simulink model "Horizontal_Turn_Symmetric"  (R2021b)
settings: Solver=ode4  StartTime=0.0  StopTime=50  FixedStep=0.01  RelTol=1e-1
values from neighbouring files (symbols this model uses):
  alpha_ = atan(y(3)/y(1))    [Trim_sym.m]    (also in Trim_sym.mat = 0.357010867724)
  b = 2.8956    [Constants_sym.m]    (also in Trim_sym_main.m)
  cbar = 0.18994    [Constants_sym.m]    (also in Trim_sym_main.m)
  Cprop = 1    [Constants_sym.m]    (also in Trim_sym_main.m)
  d2r = pi/180    (= 0.0174532925199)    [Constants_sym.m]    (also in Trim_sym.m; Trim_sym_main.m)
  g = 9.81    [Constants_sym.m]    (also in Trim_sym_main.m)
  Ixx = 0.8244    [Constants_sym.m]    (also in Trim_sym_main.m)
  Ixz = 0.1204    [Constants_sym.m]    (also in Trim_sym_main.m)
  Iyy = 1.135    [Constants_sym.m]    (also in Trim_sym_main.m)
  Izz = 1.759    [Constants_sym.m]    (also in Trim_sym_main.m)
  Kmotor = 80    [Constants_sym.m]    (also in Trim_sym_main.m)
  m = 13.5    [Constants_sym.m]    (also in Trim_sym_main.m)
  q = 0    [Trim_sym.m]
  qbar = 0.5*rho*V^2    [Constants_sym.m]    (also in Trim_sym_main.m = 186.625322459)
  r = 0    [Trim_sym.m]
  r2d = 180/pi    (= 57.2957795131)    [Constants_sym.m]    (also in Trim_sym.m; Trim_sym_main.m)
  rho = p_atm/(287*T_atm)    [Constants_sym.m]    (also in Trim_sym_main.m = 1.44533597728)
  S = 0.55    [Constants_sym.m]    (also in Trim_sym_main.m)
  Sprop = 0.2027    [Constants_sym.m]    (also in Trim_sym_main.m)
  V = 16.07    [Trim_sym.mat]    (also in Trim_sym_main.m)
undefined symbols (not defined in the file or in its folder): F, Light, MIL, sigbuilder_block
libraries: aerolibwind2 x3, simulink x1, slpidlib x1, sharedtransform x1
(part 1 of 2)
settings Model: Creator=Prateek  LastModifiedBy=piyus
settings SolverCC: MaxConsecutiveMinStep=100  AlgebraicLoopSolver=LineSearch
settings DataIOCC: ReturnWorkspaceOutputs=off
settings DebuggingCC: SFMachineParentedDataDiag=warning  ArithmeticOperatorsInVariantConditions=warning
settings SFSimCC: CustomCodeUndefinedFunction=UseInterfaceOnly

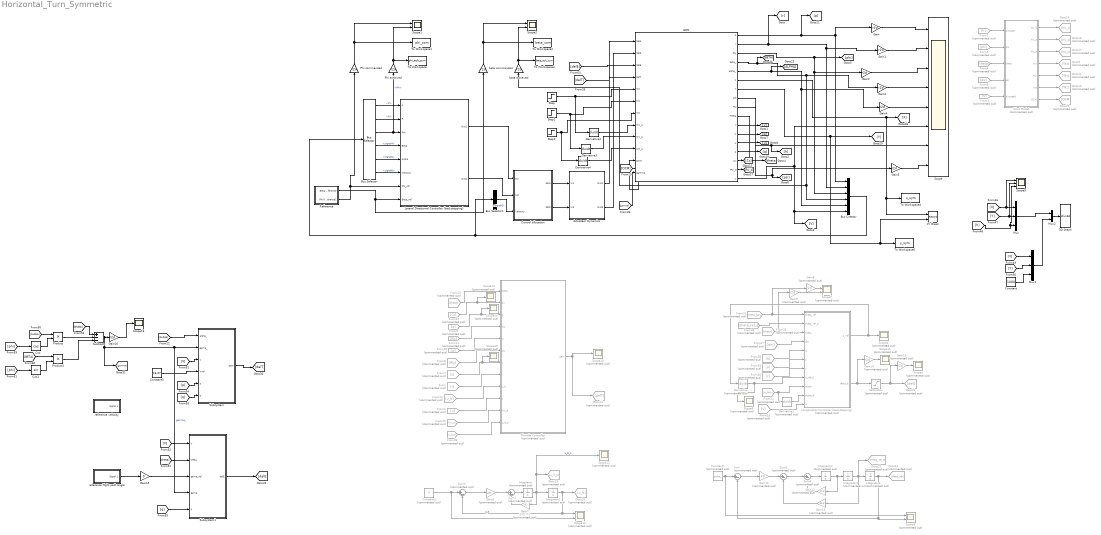
== system Horizontal_Turn_Symmetric ==
  3D Graph : S-Function  LoadFcn=if exist('sfun3d','file'), sfun3d([],[],[],'LoadBlock'); end  FunctionName=sfun3d  Parameters=ax,T,np,cp,gd,ls,mk,mx,hd,tb  SFunctionDeploymentMode=off  EnableBusSupport=off  mask(3D Graph){np=2, ax=[0 500 -20 300 500 3000], mx=1e4, T=0.01, cp=[500 -300 700], gd=on, hd=on, tb=off, ls=-, mk=.}
      mask prompts: np "Number of moving points (lines)"; ax "Range: [xmin xmax  ymin ymax zmin zmax]"; mx "Max number of points in each line"; T "Sampling Time"; cp "Camera position (use [0 0 1] for 2D XY view)"; gd "Grid (on|off)"; hd "HeadMarkers (on|off)"; tb "Toolbar (on|off)"; ls "LineStyle"; mk "LineMarker"
      mask help:
      | This block plots the position of several points in the XYZ space. The input contains the coordinates of all the points (x1,y1,z1,x2,y2,z2,...).
      | The number of moving points (lines), the XYZ ranges, sampling time, camera position, and grid (among other things) can be set as mask parameters.
      settings: CopyFcn=if exist('sfun3d','file'), sfun3d([],[],[],'CopyBlock'); end  DeleteFcn=if exist('sfun3d','file'), sfun3d([],[],[],'DeleteBlock'); end  NameChangeFcn=if exist('sfun3d','file'), sfun3d([],[],[],'NameChange'); end
      mask Help:
      | This block plots the position of several points in the XYZ space. The input contains the coordinates of all the points (x1,y1,z1,x2,y2,z2,...).
      | The number of moving points (lines), the XYZ ranges, sampling time, camera position, and grid (among other things) can be set as mask parameters.
      mask TypeOptions ls: - | -- | : | -. | none
      mask TypeOptions mk: none | . | + | o | * | x | square | diamond | v | ^ | > | < | pentagram | hexagram
      mask Display: plot([.05 .95 .95 .05 .05],[.45 .45 .95 .95 .45], 0.5+cos(0:0.1:2*pi)*0.3,0.7+sin(0:0.1:2*pi)*0.2)
  Actuataor Dynamics : Subsystem
  Bus Creator : BusCreator  Inputs=6
  Bus Selector : BusSelector  OutputSignals=P,R,Phi,signal4,signal5,signal6
  Bus Selector1 : BusSelector  OutputSignals=signal6
  Constant : Constant  Value=1000
  Constant1 : Constant  Commented=on  Value=alpha_
  Constant2 : Constant  Commented=on  Value=V
  Constant3 : Constant  Value=16.07
  Control allocation : Subsystem
  Cos : Trigonometry  Operator=cos
  Cos1 : Trigonometry
  Derivative : Derivative  Commented=on
  Derivative1 : Derivative  Commented=on
  Derivative2 : Derivative
  Derivative3 : Derivative
  Derivative4 : Derivative
  EOM : Subsystem
  From : From  Commented=on  GotoTag=r
  From1 : From  Commented=on  GotoTag=u
  From10 : From  Commented=on  GotoTag=w
  From11 : From  Commented=on  GotoTag=Wz
  From12 : From  Commented=on  GotoTag=Cx
  From13 : From  Commented=on  GotoTag=theta
  From14 : From  Commented=on  GotoTag=u_b
  From15 : From  Commented=on  GotoTag=Wx_p
  From2 : From  Commented=on  GotoTag=h
  From23 : From  Commented=on  GotoTag=u_b_p
  From24 : From  Commented=on  GotoTag=ALPHA
  From26 : From  Commented=on  GotoTag=theta
  From27 : From  Commented=on  GotoTag=phi
  From28 : From  Commented=on  GotoTag=q
  From29 : From  Commented=on  GotoTag=p
  From3 : From  Commented=on  GotoTag=V
  From30 : From  Commented=on  GotoTag=r
  From31 : From  Commented=on  GotoTag=theta_bar
  From33 : From  Commented=on  GotoTag=V
  From34 : From  Commented=on  GotoTag=theta_ref_d
  From4 : From  Commented=on  GotoTag=theta
  From5 : From  Commented=on  GotoTag=phi
  From6 : From  Commented=on  GotoTag=psi
  From7 : From  Commented=on  GotoTag=v
  From8 : From  Commented=on  GotoTag=Wy
  From9 : From  Commented=on  GotoTag=q
  Gain{,1..5,16} (7 alike) : Gain  Gain=r2d
  Gain{8..10,14} (4 alike) : Gain  Commented=on  Gain=r2d
  Gain11 : Gain  Commented=on  Gain=49
  Gain12 : Gain  Commented=on  Gain=10.8
  Gain13 : Gain  Commented=on  Gain=58.8
  Gain15 : Gain  Gain=0
  Gain6 : Gain  Commented=on  Gain=49
  Gain7 : Gain  Commented=on  Gain=2*0.7*7
  Goto11 : Goto  Commented=on  GotoTag=Wy
  Goto13 : Goto  Commented=on  GotoTag=delT
  Goto14 : Goto  Commented=on  GotoTag=Wx_p
  Goto15 : Goto  Commented=on  GotoTag=Wz
  Goto16 : Goto  Commented=on  GotoTag=Wy_p
  Goto17 : Goto  Commented=on  GotoTag=Wz_p
  Goto18 : Goto  Commented=on  GotoTag=u_b
  Goto19 : Goto  Commented=on  GotoTag=u_b_p
  Goto20 : Goto  Commented=on  GotoTag=DCM
  Goto23 : Goto  Commented=on  GotoTag=delE
  Goto24 : Goto  Commented=on  GotoTag=theta_bar
  Goto25 : Goto  Commented=on  GotoTag=theta_ref_d
  Goto9 : Goto  Commented=on  GotoTag=Wx
  Integrator{,2..4} (4 alike) : Integrator  Commented=on
  Integrator1 : Integrator  Commented=on  InitialCondition=19.5
  Lateral Directional Controller (backstepping) : Subsystem
  Longitudinal Controller (backstepping) : MATLAB Function  Commented=on  TreatAsAtomicUnit=on
  Mux : Mux  Inputs=3
  Mux1 : Mux  Inputs=3
  Mux2 : Mux  Inputs=2
  Phi acheived : Gain  Gain=r2d
  Phi commanded : Gain  Gain=r2d
  Product : Product
  Product1 : Product
  Reference : Subsystem
  Saturation : Saturate  Commented=on  UpperLimit=30*d2r  LowerLimit=-(30*d2r)
  Scope : Scope  NumInputPorts=8
  Scope1 : Scope  NumInputPorts=2
  Scope{3..4,6,10..11,13..15,19} (9 alike) : Scope  Commented=on
  Scope12 : Scope  Commented=on  NumInputPorts=2
  Scope16 : Scope
  Scope2 : Scope  NumInputPorts=2
  Scope5 : Scope  NumInputPorts=3
  Scope7 : Scope  Commented=on  NumInputPorts=2
  Scope8 : Scope  Commented=on  NumInputPorts=2
  Step : Step  Time=0  After=0  SampleTime=0
  Step1 : Step  Time=0  After=0  SampleTime=0
  Step2 : Step  Time=0  After=3  SampleTime=0
  Subsystem : Subsystem
  Subsystem1 : Subsystem
  Subtract : Sum  Inputs=+--
  Sum{,1..4} (5 alike) : Sum  Commented=on  Inputs=|+-
  Throttle Controller : Subsystem  Commented=on
  To Workspace : ToWorkspace  VariableName=phi_ach_sym  SampleTime=-1
  To Workspace1 : ToWorkspace  VariableName=phi_com  SampleTime=-1
  To Workspace2 : ToWorkspace  VariableName=beta_com  SampleTime=-1
  To Workspace3 : ToWorkspace  VariableName=beta_ach_sym  SampleTime=-1
  To Workspace4 : ToWorkspace  VariableName=x_sym  SampleTime=-1
  To Workspace5 : ToWorkspace  VariableName=y_sym  SampleTime=-1
  "Wind Model " : Subsystem  Commented=on
  XY Graph : Record  FileSettingsInternal="{\"entries\":[{\"content\":{\"excelSettings\":{\"content\":{},\"type\":\"Streamout.ExcelSettings\"}},\"type\":\"Streamout.FileSettingStorage\",\"uuid\":\"f48354ea-9da4-4102-8cec-34de0f807aaf\"}],\"packageUris\":[\"http://schema.mathworks.com/mf0/streamout_blocks/R2020a\"],\"version\":\"1.0\"}"  Layout=[1 1]  SignalsInternal="{\"entries\":[{\"content\":{\"signals\":[{\"content\":{\"blockPath\":[\"Horizontal_Turn_Symmetric/XY Graph\"],\"channel\":[],\"dimensions\":[1],\"domain\":\"Horizontal_Turn_Symmetric/XY Graph\",\"lineColor\":\"#a2142f\",\"plots\":[1],\"port\":1,\"sid\":[],\"signalID\":54,\"signalName\":\"EOM:6\"},\"type\":\"RecordBlkView.Signal\",\"uuid\":\"b83f61b6-62b6-4807-96de-0ee58c6a34da\"},{\"content\":{\"blockPath\":[\"Horizontal_Turn_Symmetric/XY Graph\"],\"channel\":[],\"dimensions\":[1],\"domain\":\"Horizontal_Turn_Symmetric/XY Graph\",\"lineColor\":\"#139fff\",\"plots\":[1],\"port\":2,\"sid\":[],\"signalID\":57,\"signalName\":\"EOM:7\"},\"type\":\"RecordBlkView.Signal\",\"uuid\":\"4337f21f-c38c-4e87-a719-4f27d7101128\"}]},\"type\":\"RecordBlkView.InputSignals\",\"uuid\":\"b9ba9dc8-fadb-49a6-9e4e-9d1384d51f42\"}],\"packageUris\":[\"http://schema.mathworks.com/mf0/streamout_blocks/R2020a\"],\"version\":\"1.0\"}"  VisualizationBindings="{\"xyplotplugin\":{\"info\":[{\"series\":[{\"bindingParametersList\":[{\"parameter\":\"X-Axis\",\"signalID\":54,\"signalName\":\"EOM:6\"},{\"parameter\":\"Y-Axis\",\"signalID\":57,\"signalName\":\"EOM:7\"}],\"seriesID\":61385}],\"subplotID\":1}]}}"  CompatibilityTag=XY  st=-1
  beta achieved : Gain  Gain=r2d
  beta commanded : Gain  Gain=r2d
  reference flight path angle : Subsystem  Tag=STV Subsys  LoadFcn=sigbuilder_block('load');  StartFcn=sigbuilder_block('start');  StopFcn=sigbuilder_block('stop');  ClipboardFcn=sigbuilder_block('clipboard');  mask(Sigbuilder block){tuvar=[0:10]}
      mask help: Simulink:masks:SigbuilderBlock_MD
      mask init:
      | if ~strcmp(get_param(bdroot(gcbh),'SimulationStatus'),'stopped') tuvar = sigbuilder_block('maskInit'); end
      settings: CopyFcn=sigbuilder_block('copy');  DeleteFcn=sigbuilder_block('delete');  ModelCloseFcn=sigbuilder_block('modelClose');  PreSaveFcn=sigbuilder_block('preSave');  PauseFcn=sigbuilder_block('pause');  ContinueFcn=sigbuilder_block('continue');  NameChangeFcn=sigbuilder_block('namechange');  OpenFcn=sigbuilder_block('open',[5.4 0 1141.2 552.6 ]);  CloseFcn=sigbuilder_block('close');
      mask Display: plot(0, 0, 100, 100,[2, 2, 32, 32, 2], [68, 8, 8, 68, 68],[32, 2], [38, 38], [32, 19, 2],[53, 60, 44], [32, 17, 17, 2],[16, 16, 31, 31]);txt = getActiveGroup(gcbh);text(2, 100, txt,'verticalAlignment', 'top');
  reference velocity : Subsystem  Tag=STV Subsys  LoadFcn=sigbuilder_block('load');  StartFcn=sigbuilder_block('start');  StopFcn=sigbuilder_block('stop');  ClipboardFcn=sigbuilder_block('clipboard');  mask(Sigbuilder block){tuvar=[0:10]}
      mask help: Simulink:masks:SigbuilderBlock_MD
      mask init:
      | if ~strcmp(get_param(bdroot(gcbh),'SimulationStatus'),'stopped') tuvar = sigbuilder_block('maskInit'); end
      settings: CopyFcn=sigbuilder_block('copy');  DeleteFcn=sigbuilder_block('delete');  ModelCloseFcn=sigbuilder_block('modelClose');  PreSaveFcn=sigbuilder_block('preSave');  PauseFcn=sigbuilder_block('pause');  ContinueFcn=sigbuilder_block('continue');  NameChangeFcn=sigbuilder_block('namechange');  OpenFcn=sigbuilder_block('open',[5.4 0 1141.2 552.6 ]);  CloseFcn=sigbuilder_block('close');
      mask Display: plot(0, 0, 100, 100,[2, 2, 32, 32, 2], [68, 8, 8, 68, 68],[32, 2], [38, 38], [32, 19, 2],[53, 60, 44], [32, 17, 17, 2],[16, 16, 31, 31]);txt = getActiveGroup(gcbh);text(2, 100, txt,'verticalAlignment', 'top');
  wires:
  Bus Creator/1 -> Bus Selector/1, Bus Selector1/1
  Control allocation/1(delA) -> Actuataor Dynamics/1(In1)
  Control allocation/2(delR) -> Actuataor Dynamics/2(In3)
  Lateral Directional Controller (backstepping)/1(Out1) -> Control allocation/1(MX)
  Phi commanded/1 -> To Workspace1/1, Scope1/1
  Lateral Directional Controller (backstepping)/2(Out2) -> Control allocation/2(MZ)
  Reference/1(Beta Reference) -> beta commanded/1, Lateral Directional Controller (backstepping)/8(Beta_ref)
  Phi acheived/1 -> Scope1/2, To Workspace/1
  beta commanded/1 -> To Workspace2/1, Scope2/1
  Gain3/1 -> Scope/4
  Gain4/1 -> Scope/5
  Gain/1 -> Scope/1
  Gain1/1 -> Scope/2
  Gain2/1 -> Scope/3
  Bus Selector1/1 -> Control allocation/3(Velocity)  "<signal6>"
  Bus Selector/1 -> Lateral Directional Controller (backstepping)/1(P)  "<P>"
  Bus Selector/2 -> Lateral Directional Controller (backstepping)/2(R)  "<R>"
  Bus Selector/3 -> Phi acheived/1, Lateral Directional Controller (backstepping)/3(PHI)  "<Phi>"
  Bus Selector/4 -> Lateral Directional Controller (backstepping)/4(Beta)  "<signal4>"
  Bus Selector/5 -> Lateral Directional Controller (backstepping)/5(Alpha)  "<signal5>"
  Bus Selector/6 -> Lateral Directional Controller (backstepping)/6(Velocity)  "<signal6>"
  Gain5/1 -> Scope/8
  Actuataor Dynamics/1(Out1) -> EOM/1(delA)
  Actuataor Dynamics/2(Out6) -> EOM/2(delR)
  [delT] -> EOM/4(delT)
  EOM/1(p) -> [p], Gain/1, Bus Creator/1
  EOM/2(r) -> Bus Creator/2, Gain1/1, [r]
  EOM/3(Phi) -> [phi], Bus Creator/3, Gain2/1
  EOM/4(beta_) -> [BETA], Bus Creator/4, beta achieved/1, Gain3/1
  EOM/5(alpha_) -> [ALPHA], Bus Creator/5, Gain4/1
  EOM/17(V) -> Scope/6, [V], Bus Creator/6
  EOM/6(X) -> [X], To Workspace4/1, XY Graph/1
  EOM/8(Alt) -> [h], Scope/7
  EOM/9(Psi) -> Gain5/1, [psi]
  beta achieved/1 -> Scope2/2, To Workspace3/1
  EOM/11(v) -> [v]
  EOM/10(Theta) -> [theta]
  EOM/12(w) -> [w]
  EOM/13(u) -> [u]
  EOM/14(q) -> [q]
  EOM/15(Cx) -> [Cx]
  From13/1 -> Throttle Controller/1(theta)
  From12/1 -> Scope14/1, Throttle Controller/2(Cx)
  From9/1 -> Scope15/1, Throttle Controller/3(q)
  From11/1 -> Throttle Controller/4(Wz)
  From10/1 -> Throttle Controller/5(w)
  From8/1 -> Throttle Controller/6(Wy)
  From7/1 -> Throttle Controller/7(v), Scope19/1
  From/1 -> Throttle Controller/8(r)
  From14/1 -> Throttle Controller/9(u_b)
  From1/1 -> Throttle Controller/10(u)
  From15/1 -> Throttle Controller/11(Wx_p)
  Throttle Controller/1(delT) -> Goto13/1, Scope10/1
  Step/1 -> Derivative2/1, EOM/5(Wx)
  Step1/1 -> Derivative3/1, EOM/6(Wy)
  Derivative2/1 -> EOM/8(Wx_p)
  Derivative3/1 -> EOM/9(Wy_p)
  Derivative4/1 -> EOM/10(Wz_p)
  Constant2/1 -> Scope12/2, Sum1/1
  Integrator1/1 -> Goto18/1, Sum1/2, Scope12/1  "u_b"
  Sum1/1 -> Gain6/1
  Gain6/1 -> Sum2/1
  Sum2/1 -> Integrator/1
  Integrator/1 -> Scope13/1, Goto19/1, Integrator1/1, Gain7/1  "u_b_p"
  Gain7/1 -> Sum2/2
  From23/1 -> Throttle Controller/12(u_b_p)
  [DCM] -> EOM/11(DCM)
  From2/1 -> "Wind Model "/1(Altitude)
  From5/1 -> "Wind Model "/2(phi)
  From4/1 -> "Wind Model "/3(theta)
  From6/1 -> "Wind Model "/4(psi)
  From3/1 -> "Wind Model "/5(Airspeed)
  "Wind Model "/1(Wx_p) -> Goto14/1
  "Wind Model "/2(Wy_p) -> Goto16/1
  "Wind Model "/3(Wz_p) -> Goto17/1
  EOM/7(Y) -> XY Graph/2, To Workspace5/1, [Y]
  "Wind Model "/4(Wx) -> Goto9/1
  "Wind Model "/5(Wy) -> Goto11/1
  "Wind Model "/6(Wz) -> Goto15/1
  "Wind Model "/7(DCM) -> Goto20/1
  From26/1 -> Longitudinal Controller (backstepping)/3(theta), Gain9/1
  From27/1 -> Longitudinal Controller (backstepping)/4(phi)
  From28/1 -> Longitudinal Controller (backstepping)/5(q)
  From29/1 -> Longitudinal Controller (backstepping)/6(p)
  From30/1 -> Longitudinal Controller (backstepping)/7(r)
  Longitudinal Controller (backstepping)/1(q_ref) -> Scope4/1, Derivative/1
  From31/1 -> Longitudinal Controller (backstepping)/1(theta_ref), Gain8/1
  From33/1 -> Longitudinal Controller (backstepping)/11(V)
  [delE] -> EOM/3(delE)
  Derivative/1 -> Scope6/1, Longitudinal Controller (backstepping)/8(q_ref_d)
  Saturation/1 -> Goto23/1, Gain10/1
  Gain9/1 -> Scope7/2
  Gain8/1 -> Scope7/1
  Gain10/1 -> Scope3/1
  Constant1/1 -> Sum/1, Scope8/1
  Integrator4/1 -> Goto24/1, Sum/2, Scope8/2
  Sum/1 -> Gain11/1
  Gain11/1 -> Sum3/1
  Sum3/1 -> Sum4/1
  Sum4/1 -> Integrator2/1
  Integrator2/1 -> Gain12/1, Integrator3/1
  Integrator3/1 -> Goto25/1, Gain13/1, Integrator4/1
  Gain12/1 -> Sum4/2
  Gain13/1 -> Sum3/2
  From34/1 -> Longitudinal Controller (backstepping)/2(theta_ref_d)
  EOM/16(Psi_d) -> [Psi_d]
  From24/1 -> Derivative1/1, Longitudinal Controller (backstepping)/9(alpha)
  Derivative1/1 -> Longitudinal Controller (backstepping)/10(alpha_d)
  Mux/1 -> Mux2/1
  [Y] -> Scope5/2, Mux/2
  [X] -> Scope5/1, Mux/1
  [h] -> Scope5/3, Mux/3
  [X] -> Mux1/1
  [Y] -> Mux1/2
  Constant/1 -> Mux1/3
  Mux1/1 -> Mux2/2
  Mux2/1 -> 3D Graph/1
  Longitudinal Controller (backstepping)/2(delta_e) -> Gain14/1, Saturation/1
  Gain14/1 -> Scope11/1
  [ALPHA] -> Subsystem/1(alpha_)
  [V] -> Subsystem/3(V)
  Subsystem/1(delT) -> [delT]
  [V] -> Subsystem1/1(V)
  [theta] -> Subsystem1/2(theta)
  [q] -> Subsystem1/5(q)
  Subsystem1/1(delE) -> [delE]
  [theta] -> Subtract/1
  [ALPHA] -> Product/1
  [p] -> Subsystem/5(p)
  [q] -> Subsystem/6(q)
  reference flight path angle/1(Signal 1) -> Gain15/1
  Cos/1 -> Product/2
  Product/1 -> Subtract/2
  [phi] -> Cos/1
  [BETA] -> Product1/1
  Cos1/1 -> Product1/2
  [phi] -> Cos1/1
  Product1/1 -> Subtract/3
  Gain16/1 -> Scope16/1
  Subtract/1 -> [gamma], Subsystem1/4(gama), Subsystem/2(gama_), Gain16/1  "gamma_"
  Gain15/1 -> Subsystem1/3(gama_ref)
  Constant3/1 -> Subsystem/4(Vref)
  [gamma] -> EOM/12(gamma)
  Reference/2(Phi Reference1) -> Phi commanded/1, Lateral Directional Controller (backstepping)/7(Phi_ref)
  Step2/1 -> Derivative4/1, EOM/7(Wz)

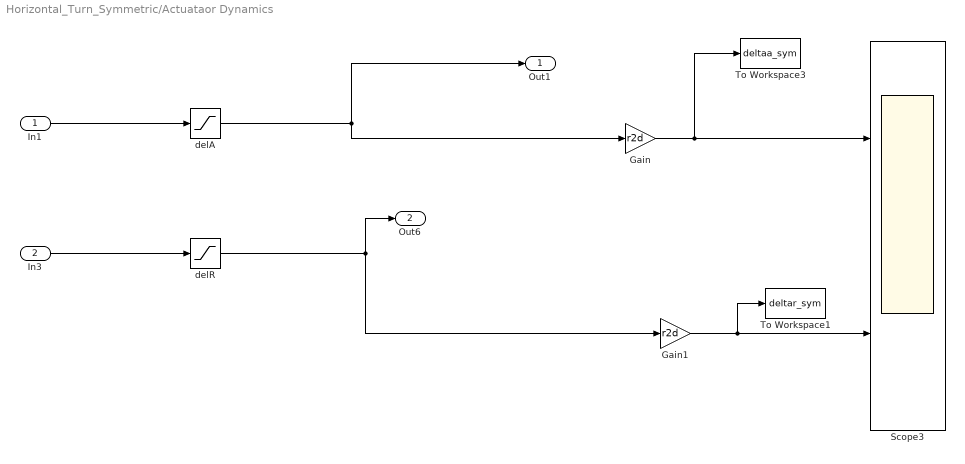
== system Horizontal_Turn_Symmetric/Actuataor Dynamics ==
  In1 : Inport
  In3 : Inport  Port=2
  Gain : Gain  Gain=r2d
  Gain1 : Gain  Gain=r2d
  Scope3 : Scope  NumInputPorts=2
  To Workspace1 : ToWorkspace  VariableName=deltar_sym  SampleTime=-1
  To Workspace3 : ToWorkspace  VariableName=deltaa_sym  SampleTime=-1
  delA : Saturate  UpperLimit=20*d2r  LowerLimit=-20*d2r
  delR : Saturate  UpperLimit=30*d2r  LowerLimit=-30*d2r
  Out1 : Outport  VectorParamsAs1DForOutWhenUnconnected=off
  Out6 : Outport  Port=2  VectorParamsAs1DForOutWhenUnconnected=off
  wires:
  delR/1 -> Gain1/1, Out6/1
  In1/1 -> delA/1
  In3/1 -> delR/1
  Gain/1 -> To Workspace3/1, Scope3/1
  Gain1/1 -> To Workspace1/1, Scope3/2
  delA/1 -> Gain/1, Out1/1

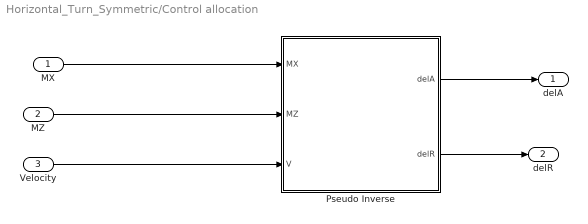
== system Horizontal_Turn_Symmetric/Control allocation ==
  MX : Inport
  MZ : Inport  Port=2
  Velocity : Inport  Port=3
  Pseudo Inverse : MATLAB Function  TreatAsAtomicUnit=on
  delA : Outport  VectorParamsAs1DForOutWhenUnconnected=off
  delR : Outport  Port=2  VectorParamsAs1DForOutWhenUnconnected=off
  wires:
  Velocity/1 -> Pseudo Inverse/3(V)
  MX/1 -> Pseudo Inverse/1(MX)
  MZ/1 -> Pseudo Inverse/2(MZ)
  Pseudo Inverse/1(delA) -> delA/1
  Pseudo Inverse/2(delR) -> delR/1

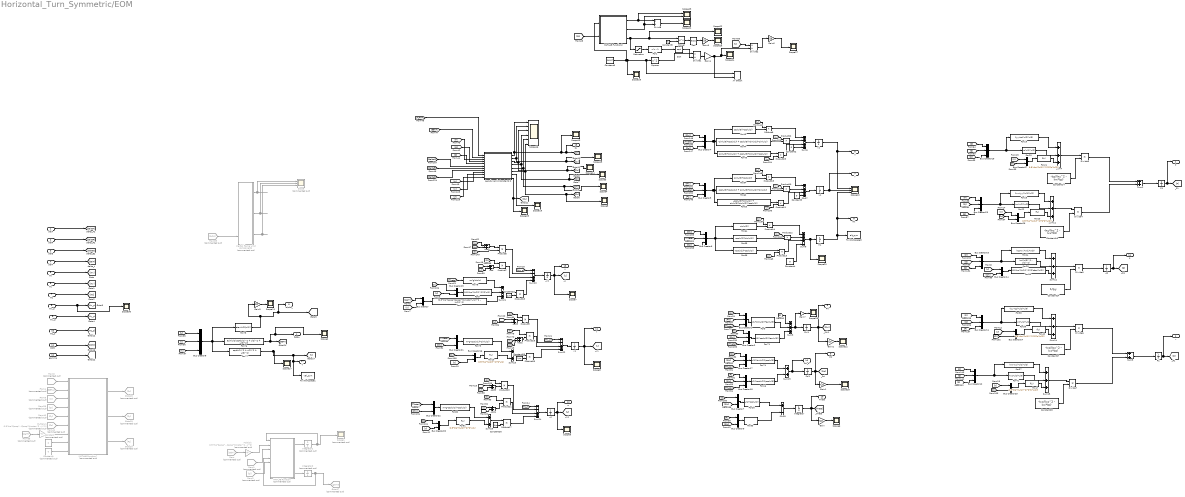
== system Horizontal_Turn_Symmetric/EOM ==
  delA : Inport
  delR : Inport  Port=2
  delE : Inport  Port=3
  delT : Inport  Port=4
  Wx : Inport  Port=5
  Wy : Inport  Port=6
  Wz : Inport  Port=7
  Wx_p : Inport  Port=8
  Wy_p : Inport  Port=9
  Wz_p : Inport  Port=10
  DCM : Inport  Port=11
  gamma : Inport  Port=12
  Add{,1..5} (6 alike) : Sum
  Aerodynamic Constants 2 : MATLAB Function  TreatAsAtomicUnit=on
  Bus Creator{,7,9,14..16,20..22,24..27} (13 alike) : BusCreator  Inputs=2
  Bus Creator{1..4,6,8,10..12,17..19,23} (13 alike) : BusCreator  Inputs=3
  Constant : Constant  Commented=on  Value=0
  Constant1 : Constant  Commented=on  Value=0
  Constant14 : Constant  Value=-Izz/(Ixz^2 - Ixx*Izz)
  Constant16 : Constant  Value=-Ixz/(Ixz^2 - Ixx*Izz)
  Constant2 : Constant  Value=0
  Constant23 : Constant  Value=1/m
  Constant24 : Constant  Value=1/Iyy
  Constant25 : Constant  Value=1/m
  Constant26 : Constant  Value=1/m
  Constant27 : Constant  Value=-Ixz/(Ixz^2 - Ixx*Izz)
  Constant28 : Constant  Value=-Ixx/(Ixz^2 - Ixx*Izz)
  Constant3 : Constant  Value=0
  Constant4 : Constant  Value=0
  Constant5 : Constant  Value=-1
  Constant6 : Constant  Value=16.07
  Cos : Trigonometry  Operator=acos
  Divide : Product  Inputs=*/
  Divide1 : Product  Inputs=*/
  Divide2 : Product  Inputs=*/
  Divide{3..7} (5 alike) : Product  Inputs=**
  Fcn1 : Fcn  Expr=u*u - 1
  Fcn10 : Fcn  Expr=0.5*rho*((u(2))^2)*S*u(1)
  Fcn16 : Fcn  Expr=u(1)*cos(u(2))/cos(u(3))
  Fcn18 : Fcn  Expr=(Ixx-Iyy)*u(1)*u(2)
  Fcn19 : Fcn  Expr=(Iyy-Izz)*u(2)*u(3)
  Fcn20 : Fcn  Expr=Ixz*u(1)*u(2)
  Fcn{21,23,40,42} (4 alike) : Fcn  Expr=0.5*rho*((u(1))^2)*S*b*(u(2))
  Fcn22 : Fcn  Expr=-Ixz*u(2)*u(3)
  Fcn24 : Fcn  Expr=(Izz-Ixx)*u(1)*u(3)
  Fcn25 : Fcn  Expr=Ixz*(u(3)^2 - u(1)^2)
  Fcn26 : Fcn  Expr=u(1)*cos(u(2))
  Fcn3 : Fcn  Expr=(0.5*rho*Sprop*Cprop)*((Kmotor*u(1))^2 - (u(2))^2)
  Fcn36 : Fcn  Expr=0.5*rho*((u(1))^2)*S*cbar*(u(2))
  Fcn37 : Fcn  Expr=(Ixx-Iyy)*u(1)*u(2)
  Fcn38 : Fcn  Expr=(Iyy-Izz)*u(2)*u(3)
  Fcn39 : Fcn  Expr=Ixz*u(1)*u(2)
  Fcn41 : Fcn  Expr=-Ixz*u(2)*u(3)
  Fcn43 : Fcn  Expr=cos(u(3))*cos(u(2))
  Fcn44 : Fcn  Expr=-sin(u(3))*cos(u(1)) + cos(u(3))*sin(u(2))*sin(u(1))
  Fcn45 : Fcn  Expr=sin(u(3))*sin(u(1)) + cos(u(3))*sin(u(2))*cos(u(1))
  Fcn5 : Fcn  Expr=0.5*rho*((u(2))^2)*S*u(1)
  Fcn53 : Fcn  Expr=u(1)*sin(u(2))
  Fcn54 : Fcn  Expr=sin(u(3))*cos(u(2))
  Fcn62 : Fcn  Expr=cos(u(3))*cos(u(1)) + sin(u(3))*sin(u(2))*sin(u(1))
  Fcn63 : Fcn  Expr=-cos(u(3))*sin(u(1)) + sin(u(3))*sin(u(2))*cos(u(1))
  Fcn64 : Fcn  Expr=sin(u(2))
  Fcn65 : Fcn  Expr=-cos(u(2))*sin(u(1))
  Fcn66 : Fcn  Expr=-cos(u(2))*cos(u(1))
  Fcn71 : Fcn  Expr=u(1)*cos(u(2))*tan(u(3))
  Fcn74 : Fcn  Expr=u(1)*sin(u(2))/cos(u(3))
  Fcn75 : Fcn  Expr=atan(u(3)/u(1))
  Fcn76 : Fcn  Expr=asin(u(2)/sqrt(u(1)^2 + u(2)^2 + u(3)^2))
  Fcn77 : Fcn  Expr=sqrt(u(1)^2 + u(2)^2 + u(3)^2)
  Fcn78 : Fcn  Expr=-m*g*sin(u)
  Fcn79 : Fcn  Expr=m*g*cos(u(1))*sin(u(2))
  Fcn80 : Fcn  Expr=m*g*cos(u(1))*cos(u(2))
  Fcn81 : Fcn  Expr=0.5*rho*((u(2))^2)*S*u(1)
  Fcn9 : Fcn  Expr=u(1)*sin(u(2))*tan(u(3))
  From : From  Commented=on  GotoTag=delT
  From1 : From  Commented=on  GotoTag=ALPHA
  From2 : From  Commented=on  GotoTag=Cl
  From3 : From  Commented=on  GotoTag=ALPHA
  From39 : From  Commented=on  GotoTag=Cx
  From4 : From  Commented=on  GotoTag=BETA
  From40 : From  Commented=on  GotoTag=Cy
  From41 : From  Commented=on  GotoTag=Cz
  From5 : From  Commented=on  GotoTag=V
  From59 : From  Commented=on  GotoTag=DCM
  From65 : From  Commented=on  GotoTag=delT
  Gain{,1..3,5..7} (7 alike) : Gain  Gain=r2d
  Gain4 : Gain  Gain=1/9.8
  Goto17 : Goto  Commented=on  GotoTag=gama
  Goto18 : Goto  Commented=on  GotoTag=Fx
  Goto19 : Goto  Commented=on  GotoTag=Fy
  Goto20 : Goto  Commented=on  GotoTag=Fz
  H1 : Integrator  InitialCondition=1000  ContinuousStateAttributes='H'
  Inertial frame wind components : MATLAB Function  Commented=on  TreatAsAtomicUnit=on
  Integrator : Integrator  InitialCondition=alpha_  ContinuousStateAttributes='THETA'
  Integrator1 : Integrator  Commented=on  InitialCondition=20
  Integrator2 : Integrator  Commented=on  InitialCondition=20
  MATLAB Function : MATLAB Function  Commented=on  TreatAsAtomicUnit=on
  MATLAB Function1 : MATLAB Function  Commented=on  TreatAsAtomicUnit=on
  MATLAB Function2 : MATLAB Function  TreatAsAtomicUnit=on
  Multiply : Gain  Commented=on  Gain=0.5*rho*Sprop*Cprop*(Kmotor^2 - V^2)
  Multiply1 : Gain  Commented=on  Gain=0.5*rho*Sprop*Cprop*(Kmotor^2 - V^2)
  P1 : Integrator  ContinuousStateAttributes='P'
  Phi1 : Integrator  ContinuousStateAttributes='PHI'
  Power : Math  Operator=pow  SaturateOnIntegerOverflow=on
  Product{6..23} (18 alike) : Product
  Psi1 : Integrator  ContinuousStateAttributes='PSI'
  R1 : Integrator  ContinuousStateAttributes='R'
  Saturation : Saturate  UpperLimit=2/sqrt(3)  LowerLimit=1
  Scope : Scope  Commented=on  NumInputPorts=3
  Scope1 : Scope  Commented=on
  Scope10 : Scope  NumInputPorts=3
  Scope{2..9,11..15,17..22,24..30} (26 alike) : Scope
  Scope16 : Scope  NumInputPorts=6
  Scope23 : Scope  NumInputPorts=2
  Sqrt : Sqrt  SaturateOnIntegerOverflow=on
  Square : Math  Operator=square  SaturateOnIntegerOverflow=on
  Sum{3..4,11..12,14..15,21} (7 alike) : Sum  Inputs=+++
  Sum{2,5,19,23,25} (5 alike) : Sum
  Sum20 : Sum  Inputs=--++
  Sum22 : Sum  Inputs=--++
  Sum24 : Sum  Inputs=--++
  Sum6 : Sum  Inputs=++++
  Sum7 : Sum  Inputs=++++
  Sum8 : Sum  Inputs=+++-
  Sum9 : Sum  Inputs=+-
  To Workspace1 : ToWorkspace  VariableName=vel_sym  SampleTime=-1
  To Workspace3 : ToWorkspace  VariableName=alt_sym  SampleTime=-1
  XY Graph : Record  FileSettingsInternal="{\"entries\":[{\"content\":{\"excelSettings\":{\"content\":{},\"type\":\"Streamout.ExcelSettings\"}},\"type\":\"Streamout.FileSettingStorage\",\"uuid\":\"0f9652c8-27f8-4f73-baa0-5938e709fb6d\"}],\"packageUris\":[\"http://schema.mathworks.com/mf0/streamout_blocks/R2020a\"],\"version\":\"1.0\"}"  Layout=[1 1]  SignalsInternal="{\"entries\":[{\"content\":{\"signals\":[{\"content\":{\"blockPath\":[\"Horizontal_Turn_Symmetric/EOM/XY Graph\"],\"channel\":[],\"dimensions\":[1],\"domain\":\"Horizontal_Turn_Symmetric/EOM/XY Graph\",\"lineColor\":\"#a2142f\",\"plots\":[1],\"port\":1,\"sid\":[],\"signalID\":62,\"signalName\":\"Constant6\"},\"type\":\"RecordBlkView.Signal\",\"uuid\":\"af1bedff-1c73-408a-b403-2aa099f34626\"},{\"content\":{\"blockPath\":[\"Horizontal_Turn_Symmetric/EOM/XY Graph\"],\"channel\":[],\"dimensions\":[1],\"domain\":\"Horizontal_Turn_Symmetric/EOM/XY Graph\",\"lineColor\":\"#139fff\",\"plots\":[1],\"port\":2,\"sid\":[],\"signalID\":65,\"signalName\":\"Gain4\"},\"type\":\"RecordBlkView.Signal\",\"uuid\":\"87c22434-c0b1-4fac-a9e5-b46ee65c5a67\"}]},\"type\":\"RecordBlkView.InputSignals\",\"uuid\":\"99e9dcdf-9075-4100-8f2a-a5126c4a73a6\"}],\"packageUris\":[\"http://schema.mathworks.com/mf0/streamout_blocks/R2020a\"],\"version\":\"1.0\"}"  VisualizationBindings="{\"xyplotplugin\":{\"info\":[{\"series\":[{\"bindingParametersList\":[{\"parameter\":\"X-Axis\",\"signalID\":62,\"signalName\":\"Constant6\"},{\"parameter\":\"Y-Axis\",\"signalID\":65,\"signalName\":\"Gain4\"}],\"seriesID\":14205}],\"subplotID\":1}]}}"  CompatibilityTag=XY  st=-1
  _Q : Integrator  ContinuousStateAttributes='Q'
  _u1 : Integrator  InitialCondition=15.06  ContinuousStateAttributes='u'
  _w : Integrator  InitialCondition=5.616  ContinuousStateAttributes='w'
  v1 : Integrator  ContinuousStateAttributes='v'
  x1 : Integrator  ContinuousStateAttributes='x'
  y1 : Integrator  ContinuousStateAttributes='y'
  p : Outport
  r : Outport  Port=2
  Phi : Outport  Port=3
  beta_ : Outport  Port=4
  alpha_ : Outport  Port=5
  X : Outport  Port=6
  Y : Outport  Port=7
  Alt : Outport  Port=8
  Psi : Outport  Port=9
  Theta : Outport  Port=10
  v : Outport  Port=11
  w : Outport  Port=12
  u : Outport  Port=13
  q : Outport  Port=14
  Cx : Outport  Port=15
  Psi_d : Outport  Port=16
  V : Outport  Port=17
  wires:
  [BETA] -> Aerodynamic Constants 2/2(beta_)
  [Theta] -> Bus Creator21/1
  Fcn54/1 -> Product19/2
  [Q] -> Bus Creator11/2
  [Phi] -> Bus Creator17/2
  delA/1 -> [deltaA]
  Sum24/1 -> _w/1  "Wdot"
  [P] -> Bus Creator19/1
  Sum8/1 -> Scope20/1, H1/1  "HDot"
  Fcn71/1 -> Sum3/3
  Phi1/1 -> Phi/1, Gain2/1, [Phi]  "Phi"
  [v] -> Product22/1
  Bus Creator18/1 -> Fcn16/1
  [Q] -> Bus Creator19/2
  Fcn40/1 -> Sum14/3
  [Phi] -> Bus Creator2/2
  Fcn20/1 -> Sum4/2
  Constant28/1 -> Divide7/2
  Product21/1 -> Sum24/3
  [Q] -> Aerodynamic Constants 2/4(Q)
  Fcn62/1 -> Product10/2
  Product13/1 -> Sum8/3
  Sum19/1 -> Psi_d/1, Psi1/1  "Psi dot"
  Fcn64/1 -> Product14/2
  Fcn18/1 -> Sum11/1
  [w] -> Add2/1
  Fcn75/1 -> alpha_/1, [ALPHA], Gain3/1
  [Theta] -> Bus Creator4/2
  Fcn42/1 -> Sum15/3
  P1/1 -> p/1, [P]  "P"
  Fcn81/1 -> Sum25/2
  Fcn10/1 -> Sum23/2
  Constant16/1 -> Divide4/2
  Bus Creator10/1 -> Fcn24/1, Fcn25/1
  [Phi] -> Bus Creator21/2
  Fcn79/1 -> Sum23/1
  Product18/1 -> Sum22/3
  Fcn9/1 -> Sum3/2
  Sum2/1 -> P1/1  "Pdot"
  Bus Creator8/1 -> Fcn77/1, Fcn75/1, Fcn76/1
  [Phi] -> Bus Creator18/2
  Divide6/1 -> Sum5/1
  Fcn80/1 -> Sum25/1
  Product22/1 -> Sum6/2
  Fcn38/1 -> Sum14/1
  Sum23/1 -> Product16/1
  Product23/1 -> Sum6/3
  Sum3/1 -> Gain7/1, Phi1/1  "Phi dot"
  Fcn24/1 -> Sum12/1
  Bus Creator12/1 -> Fcn37/1, Fcn41/1
  Constant14/1 -> Divide3/2
  [Phi] -> Bus Creator22/2
  [V] -> Bus Creator15/2
  Fcn22/1 -> Sum11/2
  _w/1 -> Scope9/1, w/1, [w]  "w"
  [Cx] -> Bus Creator15/1
  Constant23/1 -> Product15/2
  Bus Creator20/1 -> Fcn81/1
  [w] -> Product13/2
  [V] -> Bus Creator16/2
  [R] -> Bus Creator23/3
  _Q/1 -> q/1, [Q]  "Q"
  Bus Creator/1 -> Fcn3/1
  Sum11/1 -> Divide4/1
  [Cm] -> Bus Creator14/2
  Integrator/1 -> Gain/1, Theta/1, [Theta]  "heta"
  Bus Creator15/1 -> Fcn5/1
  Product15/1 -> Sum20/4
  [v] -> Product12/1
  [V] -> Bus Creator/2
  [P] -> Product18/1
  [P] -> Sum3/1
  Sum4/1 -> Divide3/1
  Sum9/1 -> Integrator/1  "Theta dot"
  [P] -> Bus Creator12/1
  [deltaR] -> Aerodynamic Constants 2/8(delR)
  Fcn74/1 -> Sum19/1
  delT/1 -> [delT]
  delE/1 -> [deltaE]
  [P] -> Bus Creator11/1
  Sum22/1 -> v1/1  "Vdot"
  [R] -> Bus Creator18/1
  [Psi] -> Bus Creator6/3
  Aerodynamic Constants 2/2(Cy) -> Scope15/1, [Cy], Scope16/2
  Fcn21/1 -> Sum4/3
  [w] -> Add1/1
  Sum7/1 -> y1/1  "YDot"
  [Phi] -> Bus Creator3/1
  [P] -> Bus Creator10/1
  [u] -> Add4/1
  [v] -> Add5/2
  Bus Creator22/1 -> Fcn80/1
  Aerodynamic Constants 2/5(Cm) -> Scope4/1, [Cm], Scope16/5
  [Theta] -> Fcn78/1
  Sum20/1 -> _u1/1  "Udot"
  Bus Creator19/1 -> Fcn19/1, Fcn20/1
  [Q] -> Bus Creator12/2
  [Q] -> Product6/2
  delR/1 -> [deltaR]
  Divide7/1 -> Sum5/2
  y1/1 -> Y/1, Scope10/2  "Y"
  [Phi] -> Bus Creator4/1
  [R] -> Aerodynamic Constants 2/5(R)
  Product7/1 -> Sum20/3
  Fcn66/1 -> Product13/1
  [Theta] -> Bus Creator18/3
  [Theta] -> Bus Creator6/2
  [u] -> Product19/1
  Aerodynamic Constants 2/4(Cl) -> Scope3/1, [Cl], Scope16/4
  Sum12/1 -> Divide5/1
  [R] -> Product7/1
  [u] -> Product14/1
  Fcn76/1 -> Scope2/1, beta_/1, [BETA]
  Product11/1 -> Sum7/3
  [Psi] -> Bus Creator3/3
  [Q] -> Bus Creator7/1
  Fcn5/1 -> Sum21/2
  [Theta] -> Bus Creator2/3
  _u1/1 -> Scope7/1, u/1, [u]  "u"
  [R] -> Bus Creator2/1
  [u] -> Add3/2
  Bus Creator3/1 -> Fcn54/1, Fcn63/1, Fcn62/1
  Fcn53/1 -> Sum9/2
  v1/1 -> Scope8/1, v/1, [v]  "v"
  Sum6/1 -> x1/1  "XDot"
  Divide5/1 -> _Q/1  "Qdot"
  Fcn45/1 -> Product23/1
  Sum5/1 -> R1/1  "Rdot"
  Aerodynamic Constants 2/1(Cx) -> Scope13/1, Cx/1, [Cx], Scope16/1
  Product17/1 -> Sum24/4
  Constant24/1 -> Divide5/2
  Fcn43/1 -> Product8/2
  Constant26/1 -> Product17/2
  Constant27/1 -> Divide6/2
  Psi1/1 -> Gain1/1, Psi/1, [Psi]  "Psi"
  H1/1 -> To Workspace3/1, Alt/1, Scope10/3  "H"
  Fcn39/1 -> Sum14/2
  [Theta] -> Bus Creator1/3
  Product8/1 -> Sum6/1
  [R] -> Product9/1
  [R] -> Bus Creator10/3
  Product20/1 -> Sum24/2
  Sum25/1 -> Product17/1
  Fcn77/1 -> To Workspace1/1, V/1, [V], Scope17/1
  Bus Creator11/1 -> Fcn38/1, Fcn39/1
  [Psi] -> Bus Creator4/3
  Divide3/1 -> Sum2/1
  [Phi] -> Bus Creator7/2
  Fcn37/1 -> Sum15/1
  [R] -> Bus Creator11/3
  [P] -> Bus Creator23/1
  [Cy] -> Bus Creator16/1
  [w] -> Aerodynamic Constants 2/11(w)
  Aerodynamic Constants 2/6(Cn) -> Scope5/1, [Cn], Scope16/6
  Bus Creator4/1 -> Fcn43/1, Fcn45/1, Fcn44/1
  [Theta] -> Bus Creator3/2
  [Phi] -> Bus Creator9/2
  [v] -> Product10/1
  [P] -> Product20/1
  [Q] -> Bus Creator17/1
  Product9/1 -> Sum22/2
  Bus Creator21/1 -> Fcn79/1
  [w] -> Product23/2
  [Q] -> Bus Creator23/2
  [R] -> Bus Creator9/1
  [R] -> Bus Creator12/3
  [Phi] -> Bus Creator1/2
  Bus Creator17/1 -> Fcn74/1
  Bus Creator7/1 -> Fcn26/1
  [deltaE] -> Aerodynamic Constants 2/7(delE)
  Product16/1 -> Sum22/4
  Bus Creator24/1 -> Fcn40/1
  [deltaA] -> Aerodynamic Constants 2/6(delA)
  Sum14/1 -> Divide6/1
  [Q] -> Bus Creator10/2
  [V] -> Bus Creator14/1
  Fcn63/1 -> Product11/1
  Bus Creator2/1 -> Fcn71/1
  [w] -> Product11/2
  [v] -> Aerodynamic Constants 2/10(v)
  Product12/1 -> Sum8/2
  Aerodynamic Constants 2/3(Cz) -> Scope14/1, [Cz], Scope16/3
  Bus Creator6/1 -> Fcn66/1, Fcn65/1, Fcn64/1
  [u] -> Aerodynamic Constants 2/9(u)
  Fcn41/1 -> Sum15/2
  Fcn65/1 -> Product12/2
  x1/1 -> Scope10/1, X/1  "X"
  Fcn26/1 -> Sum9/1
  Fcn36/1 -> Sum12/3
  [V] -> Bus Creator24/1
  Bus Creator14/1 -> Fcn36/1
  [V] -> Bus Creator26/1
  Divide4/1 -> Sum2/2
  [V] -> Bus Creator27/1
  Fcn25/1 -> Sum12/2
  Constant25/1 -> Product16/2
  Fcn44/1 -> Product22/2
  [Phi] -> Bus Creator6/1
  [V] -> Bus Creator20/2
  R1/1 -> r/1, [R]  "R"
  Bus Creator16/1 -> Fcn10/1
  Product10/1 -> Sum7/2
  Fcn3/1 -> Sum21/3
  Fcn19/1 -> Sum4/1
  Sum15/1 -> Divide7/1
  [u] -> Product8/1
  Product14/1 -> Sum8/1
  [Q] -> Product21/1
  Bus Creator27/1 -> Fcn21/1
  [Q] -> Bus Creator1/1
  Fcn78/1 -> Sum21/1
  Bus Creator1/1 -> Fcn9/1
  [Cn] -> Bus Creator25/2
  Product19/1 -> Sum7/1
  [Cn] -> Bus Creator26/2
  [Cl] -> Bus Creator24/2
  [P] -> Aerodynamic Constants 2/3(P)
  [Cl] -> Bus Creator27/2
  Fcn16/1 -> Sum19/2
  Bus Creator25/1 -> Fcn42/1
  [v] -> Add/2
  [Cz] -> Bus Creator20/1
  [ALPHA] -> Aerodynamic Constants 2/1(alpha_)
  [delT] -> Bus Creator/1
  Fcn23/1 -> Sum11/3
  Product6/1 -> Sum20/2
  Bus Creator9/1 -> Fcn53/1
  [R] -> Bus Creator19/3
  Bus Creator26/1 -> Fcn23/1
  Sum21/1 -> Product15/1
  [V] -> Bus Creator25/1
  Bus Creator23/1 -> Fcn18/1, Fcn22/1
  [Theta] -> Bus Creator17/3
  [Theta] -> Bus Creator22/1
  Wx/1 -> [Wx]
  Wy/1 -> [Wy]
  Wz/1 -> [Wz]
  Wx_p/1 -> Scope30/1, [Wx_p]
  Wy_p/1 -> [Wy_p]
  Wz_p/1 -> [Wz_p]
  [Wy] -> Add/1
  Add/1 -> Product7/2
  [Wz] -> Add1/2
  Add1/1 -> Product6/1
  [Wx_p] -> Sum20/1
  [Wz] -> Add2/2
  Add2/1 -> Product18/2
  Add3/1 -> Product9/2
  [Wx] -> Add3/1
  [Wy_p] -> Sum22/1
  [Wx] -> Add4/2
  Add4/1 -> Product21/2
  Add5/1 -> Product20/2
  [Wy] -> Add5/1
  [Wz_p] -> Sum24/1
  Inertial frame wind components/1(Wx_i) -> Scope/1
  Inertial frame wind components/2(Wy_i) -> Scope/2
  Inertial frame wind components/3(Wz_i) -> Scope/3
  Constant2/1 -> Sum6/4
  Constant3/1 -> Sum7/4
  Constant4/1 -> Sum8/4
  DCM/1 -> [DCM]
  From59/1 -> Inertial frame wind components/4(dcm)
  [u] -> Bus Creator8/1
  [v] -> Bus Creator8/2
  [w] -> Bus Creator8/3
  MATLAB Function/1(V_dot) -> Integrator1/1
  Integrator1/1 -> Scope1/1, MATLAB Function/1(V)
  From/1 -> Multiply/1
  Multiply/1 -> MATLAB Function/2(Ft)
  From1/1 -> MATLAB Function/3(alpha_)
  MATLAB Function/4(gama_dot) -> Integrator2/1
  Integrator2/1 -> Goto17/1, MATLAB Function/5(gama)
  From2/1 -> MATLAB Function/6(Cl)
  From3/1 -> MATLAB Function1/1(alpha)
  From4/1 -> MATLAB Function1/2(beta)
  From5/1 -> MATLAB Function1/3(V)
  From39/1 -> MATLAB Function1/4(Cx)
  From40/1 -> MATLAB Function1/5(Cy)
  From41/1 -> MATLAB Function1/6(Cz)
  MATLAB Function1/1(Fx) -> Goto18/1
  MATLAB Function1/2(Fy) -> Goto19/1
  MATLAB Function1/3(Fz) -> Goto20/1
  From65/1 -> Multiply1/1
  Multiply1/1 -> MATLAB Function1/7(Tx)
  Constant/1 -> MATLAB Function1/8(Ty)
  Constant1/1 -> MATLAB Function1/9(Tz)
  Gain/1 -> Scope6/1
  Gain1/1 -> Scope18/1
  Gain2/1 -> Scope12/1
  Gain3/1 -> Scope11/1
  Aerodynamic Constants 2/7(CD) -> Scope19/1
  [CL] -> MATLAB Function2/2(CL)
  MATLAB Function2/1(L) -> Scope23/1, Divide/1
  MATLAB Function2/2(W) -> Scope23/2, Divide/2
  Divide/1 -> Scope21/1  "n (load factor)"
  MATLAB Function2/3(n) -> Saturation/1, Power/1, Scope22/1
  Aerodynamic Constants 2/8(CL) -> Scope25/1, [CL]
  Fcn1/1 -> Sqrt/1
  Sqrt/1 -> Divide1/2
  Constant6/1 -> MATLAB Function2/1(V), Scope29/1, XY Graph/1, Square/1
  Square/1 -> Divide1/1
  Divide1/1 -> Gain4/1
  Gain4/1 -> XY Graph/2, Divide2/2, Scope24/1
  Saturation/1 -> Fcn1/1
  Cos/1 -> Gain5/1
  Gain5/1 -> Scope26/1
  Power/1 -> Cos/1
  Constant5/1 -> Power/2
  [V] -> Divide2/1
  Divide2/1 -> Gain6/1
  Gain6/1 -> Scope27/1
  gamma/1 -> [gamma]
  Gain7/1 -> Scope28/1

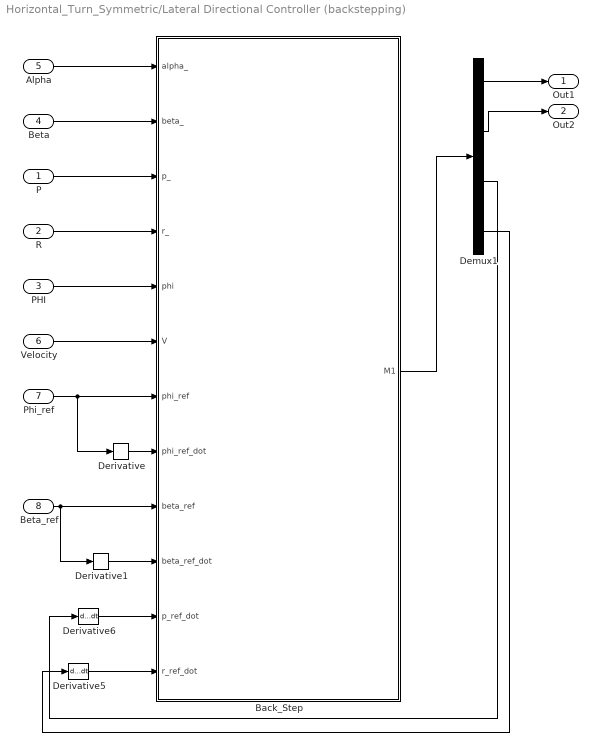
== system Horizontal_Turn_Symmetric/Lateral Directional Controller (backstepping) ==
  P : Inport
  R : Inport  Port=2
  PHI : Inport  Port=3
  Beta : Inport  Port=4
  Alpha : Inport  Port=5
  Velocity : Inport  Port=6
  Phi_ref : Inport  Port=7
  Beta_ref : Inport  Port=8
  Back_Step : MATLAB Function  TreatAsAtomicUnit=on
  Demux1 : Demux
  Derivative{,1,5..6} (4 alike) : Derivative
  Out1 : Outport  VectorParamsAs1DForOutWhenUnconnected=off
  Out2 : Outport  Port=2  VectorParamsAs1DForOutWhenUnconnected=off
  wires:
  Phi_ref/1 -> Back_Step/7(phi_ref), Derivative/1
  Derivative6/1 -> Back_Step/11(p_ref_dot)
  R/1 -> Back_Step/4(r_)
  Derivative/1 -> Back_Step/8(phi_ref_dot)
  Velocity/1 -> Back_Step/6(V)
  Alpha/1 -> Back_Step/1(alpha_)
  P/1 -> Back_Step/3(p_)
  Derivative5/1 -> Back_Step/12(r_ref_dot)
  PHI/1 -> Back_Step/5(phi)
  Back_Step/1(M1) -> Demux1/1
  Demux1/1 -> Out1/1
  Demux1/2 -> Out2/1
  Demux1/3 -> Derivative6/1
  Demux1/4 -> Derivative5/1
  Beta_ref/1 -> Derivative1/1, Back_Step/9(beta_ref)
  Derivative1/1 -> Back_Step/10(beta_ref_dot)
  Beta/1 -> Back_Step/2(beta_)

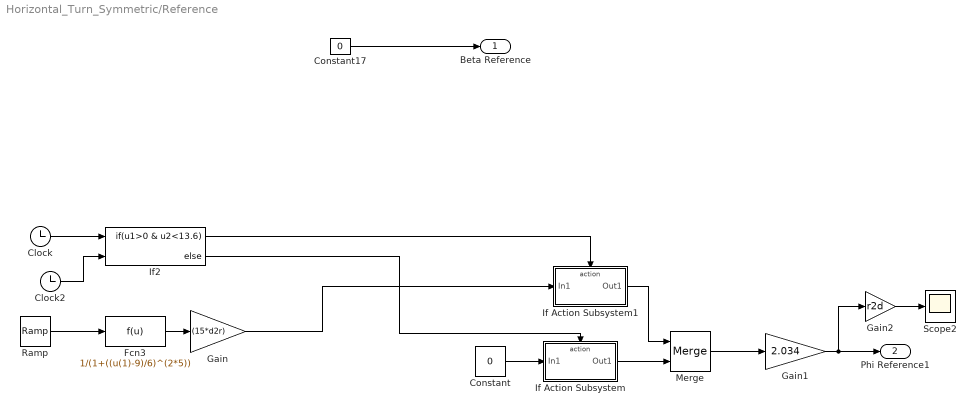
== system Horizontal_Turn_Symmetric/Reference ==
  Clock : Clock
      settings: Decimation=20
  Clock2 : Clock
      settings: Decimation=20
  Constant : Constant  Value=0
  Constant17 : Constant  Value=0
  Fcn3 : Fcn  Expr=1/(1+((u(1)-9)/6)^(2*5))
  Gain : Gain  Gain=(15*d2r)
  Gain1 : Gain  Gain=2.034
  Gain2 : Gain  Gain=r2d
  If Action Subsystem : Subsystem  TreatAsAtomicUnit=on
  If Action Subsystem1 : Subsystem  TreatAsAtomicUnit=on
  If2 : If  NumInputs=2  IfExpression=u1>0 & u2<13.6
  Merge : Merge
  Ramp : simulink/Sources/Ramp  slope=1.323  start=0  InitialOutput=0
  Scope2 : Scope
  Beta Reference : Outport  VectorParamsAs1DForOutWhenUnconnected=off
  Phi Reference1 : Outport  Port=2  VectorParamsAs1DForOutWhenUnconnected=off
  wires:
  Constant17/1 -> Beta Reference/1
  Gain/1 -> If Action Subsystem1/1(In1)
  If2/2 -> If Action Subsystem/Action
  If Action Subsystem/1(Out1) -> Merge/2
  If Action Subsystem1/1(Out1) -> Merge/1
  Gain1/1 -> Gain2/1, Phi Reference1/1
  Merge/1 -> Gain1/1
  Clock2/1 -> If2/2
  Fcn3/1 -> Gain/1
  If2/1 -> If Action Subsystem1/Action
  Constant/1 -> If Action Subsystem/1(In1)
  Ramp/1 -> Fcn3/1
  Clock/1 -> If2/1
  Gain2/1 -> Scope2/1

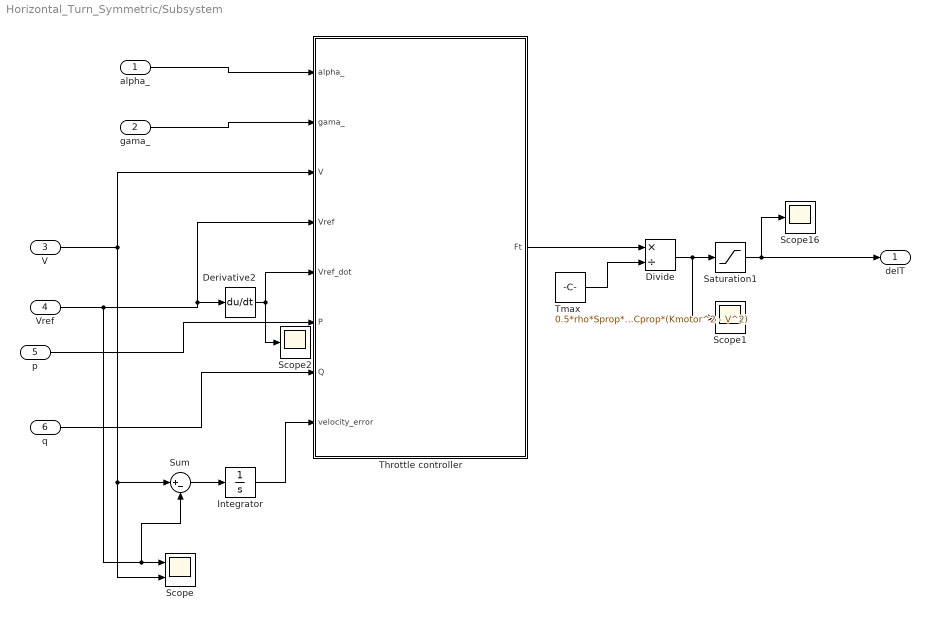
== system Horizontal_Turn_Symmetric/Subsystem ==
  alpha_ : Inport
  gama_ : Inport  Port=2
  V : Inport  Port=3
  Vref : Inport  Port=4
  p : Inport  Port=5
  q : Inport  Port=6
  Derivative2 : Derivative
  Divide : Product  Inputs=*/
  Integrator : Integrator
  Saturation1 : Saturate  UpperLimit=1  LowerLimit=0
  Scope : Scope  NumInputPorts=2
  Scope1 : Scope
  Scope16 : Scope
  Scope2 : Scope
  Sum : Sum  Inputs=|+-
  Throttle controller : MATLAB Function  TreatAsAtomicUnit=on
  Tmax : Constant  Value=0.5*rho*Sprop*Cprop*(Kmotor^2 - V^2)
  delT : Outport
  wires:
  Saturation1/1 -> delT/1, Scope16/1
  Derivative2/1 -> Scope2/1, Throttle controller/5(Vref_dot)
  gama_/1 -> Throttle controller/2(gama_)
  Divide/1 -> Scope1/1, Saturation1/1
  Vref/1 -> Sum/2, Scope/1, Derivative2/1, Throttle controller/4(Vref)
  Tmax/1 -> Divide/2
  V/1 -> Sum/1, Scope/2, Throttle controller/3(V)
  alpha_/1 -> Throttle controller/1(alpha_)
  Throttle controller/1(Ft) -> Divide/1
  p/1 -> Throttle controller/6(P)
  q/1 -> Throttle controller/7(Q)
  Sum/1 -> Integrator/1
  Integrator/1 -> Throttle controller/8(velocity_error)

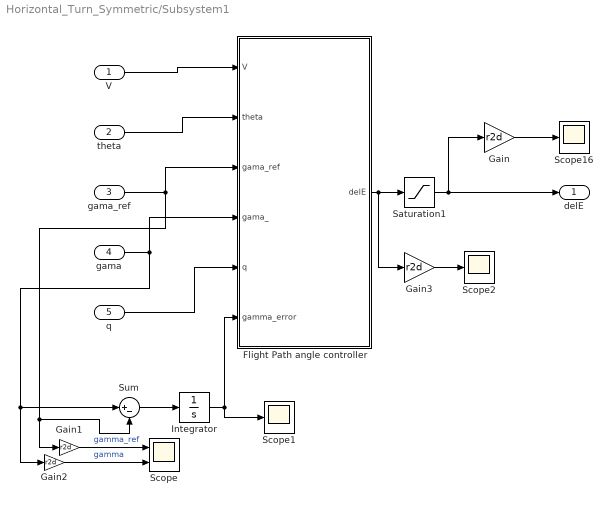
== system Horizontal_Turn_Symmetric/Subsystem1 ==
  V : Inport
  theta : Inport  Port=2
  gama_ref : Inport  Port=3
  gama : Inport  Port=4
  q : Inport  Port=5
  Flight Path angle controller : MATLAB Function  TreatAsAtomicUnit=on
  Gain{,1..3} (4 alike) : Gain  Gain=r2d
  Integrator : Integrator
  Saturation1 : Saturate  UpperLimit=30*d2r  LowerLimit=-(30*d2r)
  Scope : Scope  NumInputPorts=2
  Scope1 : Scope
  Scope16 : Scope
  Scope2 : Scope
  Sum : Sum  Inputs=|+-
  delE : Outport
  wires:
  theta/1 -> Flight Path angle controller/2(theta)
  Saturation1/1 -> delE/1, Gain/1
  Flight Path angle controller/1(delE) -> Gain3/1, Saturation1/1
  gama_ref/1 -> Sum/2, Gain1/1, Flight Path angle controller/3(gama_ref)
  q/1 -> Flight Path angle controller/5(q)
  gama/1 -> Sum/1, Gain2/1, Flight Path angle controller/4(gama_)
  V/1 -> Flight Path angle controller/1(V)
  Gain/1 -> Scope16/1
  Gain1/1 -> Scope/1  "gamma_ref"
  Gain2/1 -> Scope/2  "gamma"
  Sum/1 -> Integrator/1
  Integrator/1 -> Flight Path angle controller/6(gamma_error), Scope1/1
  Gain3/1 -> Scope2/1

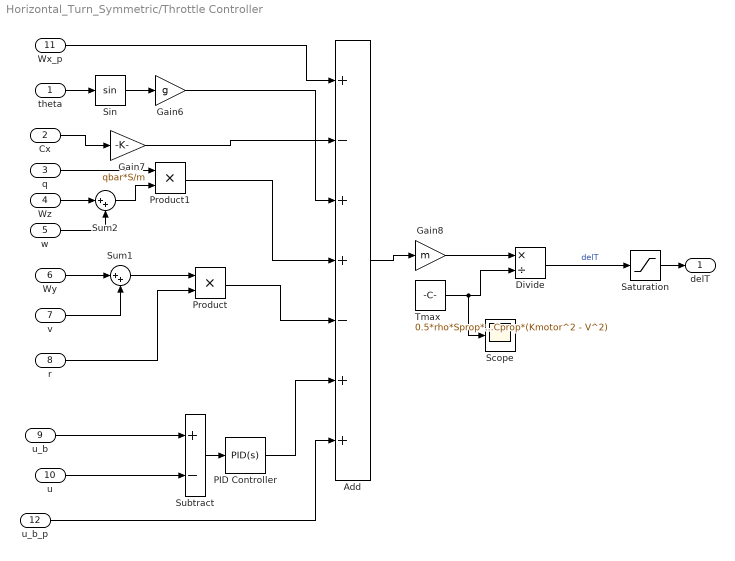
== system Horizontal_Turn_Symmetric/Throttle Controller ==
  theta : Inport
  Cx : Inport  Port=2
  q : Inport  Port=3
  Wz : Inport  Port=4
  w : Inport  Port=5
  Wy : Inport  Port=6
  v : Inport  Port=7
  r : Inport  Port=8
  u_b : Inport  Port=9
  u : Inport  Port=10
  Wx_p : Inport  Port=11
  u_b_p : Inport  Port=12
  Add : Sum  Inputs=+-++-++
  Divide : Product  Inputs=*/
  Gain6 : Gain  Gain=g
  Gain7 : Gain  Gain=qbar*S/m
  Gain8 : Gain  Gain=m
  PID Controller : slpidlib/PID Controller  Controller=PID  Form=Parallel  TimeDomain=Continuous-time  UseExternalTs=off  SampleTime=-1  IntegratorMethod=Forward Euler  FilterMethod=Forward Euler  ControllerParametersSource=internal  P=80  I=0  D=0  UseFilter=on  N=100  TunerSelectOption=Transfer Function Based (PID Tuner App)  InitialConditionSource=internal  InitialConditionForIntegrator=0  InitialConditionForFilter=0  DifferentiatorICPrevScaledInput=0  ExternalReset=none  TrackingMode=off  Kt=1  LimitOutput=off  SatLimitsSource=internal  UpperSaturationLimit=inf  LowerSaturationLimit=-inf  LinearizeAsGain=on  AntiWindupMode=none  Kb=1  POutMin=[]  POutMax=[]  IOutMin=[]  IOutMax=[]  DOutMin=[]  DOutMax=[]  NOutMin=[]  NOutMax=[]  SumOutMin=[]  SumOutMax=[]  SaturationOutMin=[]  SaturationOutMax=[]  PParamMin=[]  PParamMax=[]  IParamMin=[]  IParamMax=[]  DParamMin=[]  DParamMax=[]  NParamMin=[]  NParamMax=[]  KbParamMin=[]  KbParamMax=[]  KtParamMin=[]  KtParamMax=[]  KbOutMin=[]  KbOutMax=[]  KtOutMin=[]  KtOutMax=[]  IntegratorOutMin=[]  IntegratorOutMax=[]  FilterOutMin=[]  FilterOutMax=[]  SumI1OutMin=[]  SumI1OutMax=[]  SumI2OutMin=[]  SumI2OutMax=[]  SumI3OutMin=[]  SumI3OutMax=[]  SumI4OutMin=[]  SumI4OutMax=[]  SumDOutMin=[]  SumDOutMax=[]  DifferentiatorOutMin=[]  DifferentiatorOutMax=[]  FilterDiffOutCoefMin=[]  FilterDiffOutCoefMax=[]  ReciprocalOutMin=[]  ReciprocalOutMax=[]  SumDenOutMin=[]  SumDenOutMax=[]  SumNumOutMin=[]  SumNumOutMax=[]  DivideOutMin=[]  DivideOutMax=[]  UdiffTsProdOutMin=[]  UdiffTsProdOutMax=[]  NTsProdOutMin=[]  NTsProdOutMax=[]  UintegralTsProdOutMin=[]  UintegralTsProdOutMax=[]  UngainTsProdOutMin=[]  UngainTsProdOutMax=[]  IntegratorContinuousStateAttributes=''  IntegratorStateMustResolveToSignalObject=off  IntegratorRTWStateStorageClass=Auto  FilterContinuousStateAttributes=''  FilterStateMustResolveToSignalObject=off  FilterRTWStateStorageClass=Auto  ParallelPVariant=InternalParameters  IdealPVariant=Disabled  IVariant=InternalParameters  DVariant=InternalParameters  IntegratorVariant=Continuous  SatVariant=Disabled  AWVariant=Passthrough  PCopyVariant=Disabled  TRVariant=Disabled  FdbkBlocksVariant=Forward  IdealPFdbkVariant=Disabled  SatFdbkVariant=Disabled  DerivativeFilterVariant=ContFilter  NVariant=InternalParameters  NCopyVariant=Disabled  FilterICVariant=InternalICsFilter  IntegratorICVariant=InternalICs  ExternalResetVariant=Disabled  TRSumVariant=Passthrough  SumFdbkVariant=Disabled  SumVariant=Sum_PID  TsampFilterVariant=InternalTs  TsampNgainVariant=Passthrough  TsampIntegralVariant=Passthrough  ExternalSaturationOutDataTypeStr=Inherit: Same as second input
  Product : Product
  Product1 : Product
  Saturation : Saturate  UpperLimit=1  LowerLimit=0
  Scope : Scope
  Sin : Trigonometry
  Subtract : Sum  Inputs=+-
  Sum1 : Sum  Inputs=|++
  Sum2 : Sum  Inputs=|++
  Tmax : Constant  Value=0.5*rho*Sprop*Cprop*(Kmotor^2 - V^2)
  delT : Outport
  wires:
  u_b/1 -> Subtract/1
  PID Controller/1 -> Add/6
  Sum2/1 -> Product1/2
  Subtract/1 -> PID Controller/1
  Sum1/1 -> Product/1
  Sin/1 -> Gain6/1
  Wz/1 -> Sum2/1
  w/1 -> Sum2/2
  Product/1 -> Add/5
  Product1/1 -> Add/4
  Add/1 -> Gain8/1
  Tmax/1 -> Scope/1, Divide/2
  Gain7/1 -> Add/2
  Gain6/1 -> Add/3
  Gain8/1 -> Divide/1
  r/1 -> Product/2
  theta/1 -> Sin/1
  q/1 -> Product1/1
  Cx/1 -> Gain7/1
  u/1 -> Subtract/2
  v/1 -> Sum1/2
  Divide/1 -> Saturation/1  "delT"
  Wy/1 -> Sum1/1
  Wx_p/1 -> Add/1
  u_b_p/1 -> Add/7
  Saturation/1 -> delT/1

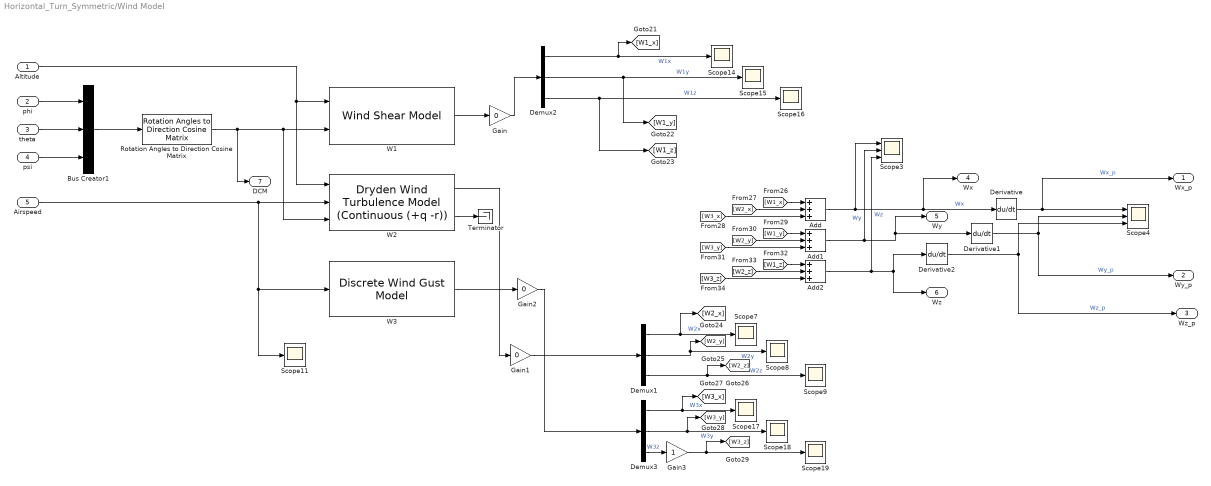
== system Horizontal_Turn_Symmetric/Wind Model  ==
  Altitude : Inport
  phi : Inport  Port=2
  theta : Inport  Port=3
  psi : Inport  Port=4
  Airspeed : Inport  Port=5
  Add : Sum  Inputs=+++
  Add1 : Sum  Inputs=+++
  Add2 : Sum  Inputs=+++
  Bus Creator1 : BusCreator  Inputs=3
  Demux1 : Demux  Outputs=3
  Demux2 : Demux  Outputs=3
  Demux3 : Demux  Outputs=3
  Derivative : Derivative
  Derivative1 : Derivative
  Derivative2 : Derivative
  Gain : Gain  Gain=0
  Gain1 : Gain  Gain=0
  Gain2 : Gain  Gain=0
  Gain3 : Gain
  Rotation Angles to Direction Cosine Matrix : sharedtransform/Rotation Angles to Direction Cosine Matrix  rotationOrder=XYZ  aMode=aMode
      settings: SourceProductBaseCode=AE,PW,DR,MT,UV,VE
  Scope{7..9,11,14..19} (10 alike) : Scope
  Scope3 : Scope  NumInputPorts=3
  Scope4 : Scope  NumInputPorts=3
  Terminator : Terminator
  W1 : aerolibwind2/Wind Shear Model  units=Metric (MKS)  phase=Category C - Terminal Flight Phase  W_20=3  Wdeg=0
  W2 : aerolibwind2/Dryden Wind Turbulence Model  (Continuous (+q -r))  units=Metric (MKS)  spec=MIL-F-8785C  model=Continuous Dryden (+q +r)  W20=0.3  Wdeg=0  TurbProb=10^-2 - Light  L_high=533  Wingspan=b  ts=0.01  Seed=[23341 23342 23343 23344]  T_on=on
  W3 : aerolibwind2/Discrete Wind Gust Model  units=Metric (MKS)  Gx=on  Gy=on  Gz=on  t_0=3  d_m=[20 30 10]  v_m=[1.5 2.5 2]
  Wx_p : Outport
  Wy_p : Outport  Port=2
  Wz_p : Outport  Port=3
  Wx : Outport  Port=4
  Wy : Outport  Port=5
  Wz : Outport  Port=6
  DCM : Outport  Port=7
  wires:
  Rotation Angles to Direction Cosine Matrix/1 -> DCM/1, W2/3, W1/2
  Derivative/1 -> Wx_p/1, Scope4/1  "Wx_p"
  Bus Creator1/1 -> Rotation Angles to Direction Cosine Matrix/1
  Demux1/1 -> [W2_x], Scope7/1  "W2x"
  Demux1/2 -> [W2_y], Scope8/1  "W2y"
  Demux2/1 -> [W1_x], Scope14/1  "W1x"
  Derivative2/1 -> Wz_p/1, Scope4/3  "Wz_p"
  W2/1 -> Gain1/1
  [W1_z] -> Add2/1
  Airspeed/1 -> W2/2, Scope11/1, W3/1
  Add/1 -> Scope3/1, Wx/1, Derivative/1  "Wx"
  Add2/1 -> Scope3/3, Wz/1, Derivative2/1  "Wz"
  [W3_x] -> Add/3
  Demux3/2 -> [W3_y], Scope18/1  "W3y"
  Demux3/1 -> Scope17/1, [W3_x]  "W3x"
  Demux2/2 -> [W1_y], Scope15/1  "W1y"
  Altitude/1 -> W2/1, W1/1
  [W3_y] -> Add1/3
  Demux2/3 -> Scope16/1, [W1_z]  "W1z"
  Add1/1 -> Scope3/2, Wy/1, Derivative1/1  "Wy"
  theta/1 -> Bus Creator1/2
  [W1_x] -> Add/1
  Demux1/3 -> [W2_z], Scope9/1  "W2z"
  [W1_y] -> Add1/1
  phi/1 -> Bus Creator1/1
  [W2_y] -> Add1/2
  [W2_z] -> Add2/2
  [W2_x] -> Add/2
  W3/1 -> Gain2/1
  Demux3/3 -> Gain3/1  "W3z"
  Derivative1/1 -> Wy_p/1, Scope4/2  "Wy_p"
  [W3_z] -> Add2/3
  psi/1 -> Bus Creator1/3
  W1/1 -> Gain/1
  W2/2 -> Terminator/1
  Gain/1 -> Demux2/1
  Gain1/1 -> Demux1/1
  Gain2/1 -> Demux3/1
  Gain3/1 -> [W3_z], Scope19/1

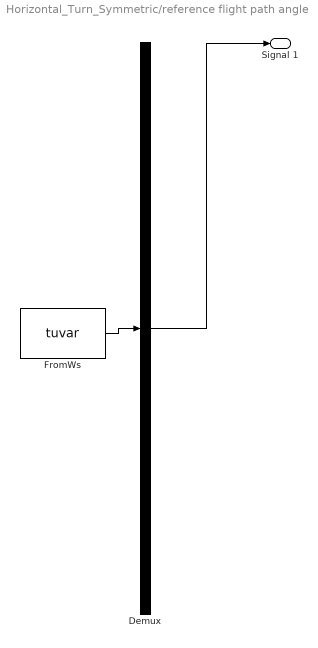
== system Horizontal_Turn_Symmetric/reference flight path angle ==
  Demux : Demux  Tag=STV Demux  Outputs=1
      settings: DisplayOption=none
  FromWs : FromWorkspace  Tag=STV FromWs  VariableName=tuvar
      SigBuilderData=|
      | common.afterFinalStr = 'Extrapolate'
      | common.sampleTime = 0
      | dataSet.timeRange = [0 10]
      | dataSet.name = 'Group 1'
      | sbobj.Groups.Name = 'Group 1'
      | sbobj.Groups.Signals.Name = 'Signal 1'
      | sbobj.Groups.Signals.XData = [0 1 5 10]
      | sbobj.Groups.Signals.YData = [0 0 0.1 0.1]
  Signal 1 : Outport  Tag=STV Outport
  wires:
  Demux/1 -> Signal 1/1
  FromWs/1 -> Demux/1

== system Horizontal_Turn_Symmetric/reference velocity ==
  Demux : Demux  Tag=STV Demux  Outputs=1
      settings: DisplayOption=none
  FromWs : FromWorkspace  Tag=STV FromWs  VariableName=tuvar
      SigBuilderData=|
      | common.afterFinalStr = 'Extrapolate'
      | common.sampleTime = 0
      | dataSet.timeRange = [0 10]
      | dataSet.name = 'Group 1'
      | sbobj.Groups.Name = 'Group 1'
      | sbobj.Groups.Signals.Name = 'Signal 1'
      | sbobj.Groups.Signals.XData = [0 4 4 10]
      | sbobj.Groups.Signals.YData = [20 20 22 22]
  Signal 1 : Outport  Tag=STV Outport
  wires:
  Demux/1 -> Signal 1/1
  FromWs/1 -> Demux/1

== system Horizontal_Turn_Symmetric/Reference/If Action Subsystem ==
  In1 : Inport
  Action Port : ActionPort  ActionPortLabel=else
  Out1 : Outport  VectorParamsAs1DForOutWhenUnconnected=off
  wires:
  In1/1 -> Out1/1

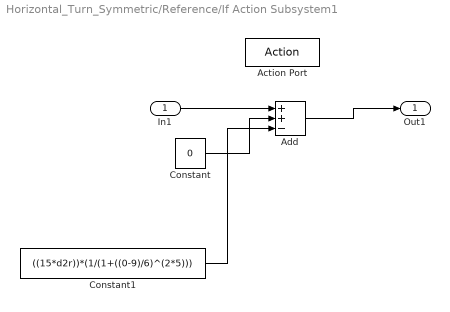
== system Horizontal_Turn_Symmetric/Reference/If Action Subsystem1 ==
  In1 : Inport
  Action Port : ActionPort  ActionPortLabel=if(u1>0 & u2<13.6)
  Add : Sum  Inputs=++-
  Constant : Constant  Value=0
  Constant1 : Constant  Value=((15*d2r))*(1/(1+((0-9)/6)^(2*5)))
  Out1 : Outport  VectorParamsAs1DForOutWhenUnconnected=off
  wires:
  In1/1 -> Add/1
  Constant/1 -> Add/2
  Add/1 -> Out1/1
  Constant1/1 -> Add/3
